simulink model "ProcNavNode"  (R2020a)
settings: Solver=FixedStepAuto  StartTime=0.0  StopTime=inf  FixedStep=.05  RelTol=1e-3
model workspace (MAT data in the model file):
  SL_ROS_VariableLengthArrays_MaxSizes.CommonInfo.ArrayTruncateAction = 'EmitWarning'
  SL_ROS_VariableLengthArrays_MaxSizes.MsgTypeMap = containers.Map
  SL_ROS_VariableLengthArrays_MaxSizes.MsgTypeMap.serialization.keys = {}
  SL_ROS_VariableLengthArrays_MaxSizes.MsgTypeMap.serialization.values = {}
  SL_ROS_VariableLengthArrays_MaxSizes.MsgTypeMap.serialization.uniformity = 0
  SL_ROS_VariableLengthArrays_MaxSizes.MsgTypeMap.serialization.keyType = 'char'
  SL_ROS_VariableLengthArrays_MaxSizes.MsgTypeMap.serialization.valueType = 'any'
libraries: robotlib x4
settings Model: SimulationMode=external  PauseTimes=1000  Creator=Lamarre  LastModifiedBy=lamarre
settings OptimizationCC: EnhancedBackFolding=on  PassReuseOutputArgsAs=Individual arguments  ZeroExternalMemoryAtStartup=off  ZeroInternalMemoryAtStartup=off  MaxStackSize=64  OptimizeBlockOrder=speed  DifferentSizesBufferReuse=on  OptimizationCustomize=off  EfficientTunableParamExpr=on
settings DebuggingCC: ParameterTunabilityLossMsg=error  FcnCallInpInsideContextMsg=warning  UnderSpecifiedDimensionMsg=warning
settings HardwareCC: ProdBitPerPointer=32  ProdBitPerSizeT=32  ProdBitPerPtrDiffT=32  ProdLargestAtomicInteger=Long  ProdWordSize=32  ProdHWDeviceType=ARM Compatible->ARM 8
settings ModelReferenceCC: ModelReferenceNumInstancesAllowed=Single
settings SFSimCC: MATLABDynamicMemAlloc=off
settings RTWCC: SystemTargetFile=ert.tlc  HardwareBoard=Robot Operating System (ROS)  TemplateMakefile=ert_default_tmf  Toolchain=Catkin  BuildConfiguration=Faster Runs  TargetLang=C++
settings CodeAppCC: ForceParamTrailComments=on  IgnoreCustomStorageClasses=off  OperatorAnnotations=on  SimulinkDataObjDesc=on  SFDataObjDesc=on  InsertBlockDesc=on
settings ERTTargetCC: MultiInstanceERTCode=on  CodeInterfacePackaging=C++ class  RootIOFormat=Structure reference

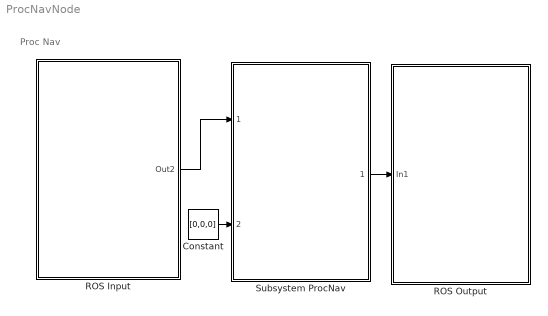
== system ProcNavNode ==
  note: Proc Nav
  Constant : Constant  Value=[0,0,0]
  ROS Input : Subsystem
  ROS Output : Subsystem
  Subsystem ProcNav : Subsystem  ReferencedSubsystem=ProcNav
  wires:
  ROS Input/1(Out2) -> Subsystem ProcNav/1
  Subsystem ProcNav/1 -> ROS Output/1(In1)
  Constant/1 -> Subsystem ProcNav/2

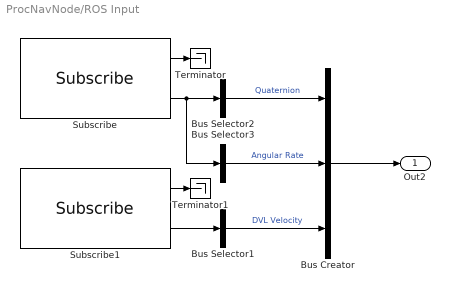
== system ProcNavNode/ROS Input ==
  Bus Creator : BusCreator  Inputs=3
  Bus Selector1 : BusSelector  OutputSignals=XVelBtm,YVelBtm,ZVelBtm  OutputAsBus=on
  Bus Selector2 : BusSelector  OutputSignals=Orientation.W,Orientation.X,Orientation.Y,Orientation.Z  OutputAsBus=on
  Bus Selector3 : BusSelector  OutputSignals=AngularVelocity.X,AngularVelocity.Y,AngularVelocity.Z  OutputAsBus=on
  Subscribe : robotlib/Subscribe  topicSource=Specify your own  topic=/provider_imu/imu_info  messageType=sensor_msgs/Imu  sampleTime=-1  messageQueueLength=1
  Subscribe1 : robotlib/Subscribe  topicSource=Specify your own  topic=/provider_dvl/dvl_velocity  messageType=sonia_common/BodyVelocityDVL  sampleTime=-1  messageQueueLength=1
  Terminator : Terminator
  Terminator1 : Terminator
  Out2 : Outport
  wires:
  Bus Selector3/1 -> Bus Creator/2  "Angular Rate"
  Bus Selector1/1 -> Bus Creator/3  "DVL Velocity"
  Bus Creator/1 -> Out2/1
  Subscribe1/1 -> Terminator1/1
  Subscribe/1 -> Terminator/1
  Bus Selector2/1 -> Bus Creator/1  "Quaternion"
  Subscribe/2 -> Bus Selector3/1, Bus Selector2/1
  Subscribe1/2 -> Bus Selector1/1

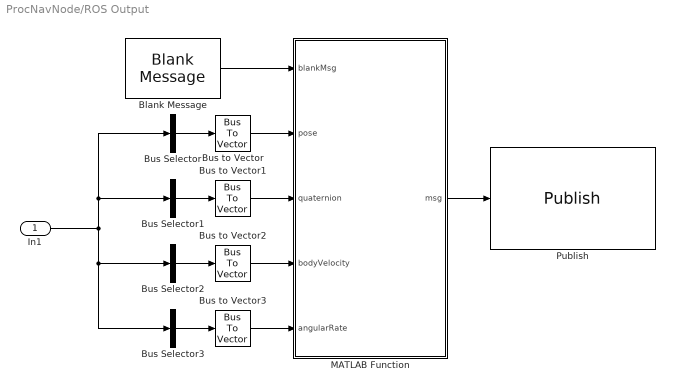
== system ProcNavNode/ROS Output ==
  In1 : Inport
  Blank Message : robotlib/Blank Message  messageClass=Message  entityType=sonia_common/ControllerStates  messageType=sonia_common/ControllerStates  SampleTime=inf
  Bus Selector : BusSelector  OutputSignals=World Position  OutputAsBus=on
  Bus Selector1 : BusSelector  OutputSignals=qS2W  OutputAsBus=on
  Bus Selector2 : BusSelector  OutputSignals=Body Velocity  OutputAsBus=on
  Bus Selector3 : BusSelector  OutputSignals=Angular Rate  OutputAsBus=on
  Bus to Vector{,1..3} (4 alike) : BusToVector
  MATLAB Function : MATLAB Function  TreatAsAtomicUnit=on
  Publish : robotlib/Publish  topicSource=Specify your own  topic=/proc_control/mesured_output  messageType=sonia_common/ControllerStates  messageQueueLength=1
  wires:
  Bus to Vector/1 -> MATLAB Function/2(pose)
  Bus to Vector2/1 -> MATLAB Function/4(bodyVelocity)
  Bus Selector2/1 -> Bus to Vector2/1
  Bus to Vector1/1 -> MATLAB Function/3(quaternion)
  In1/1 -> Bus Selector3/1, Bus Selector2/1, Bus Selector1/1, Bus Selector/1
  Blank Message/1 -> MATLAB Function/1(blankMsg)
  Bus Selector1/1 -> Bus to Vector1/1
  Bus to Vector3/1 -> MATLAB Function/5(angularRate)
  MATLAB Function/1(msg) -> Publish/1
  Bus Selector/1 -> Bus to Vector/1
  Bus Selector3/1 -> Bus to Vector3/1

== matlab function ProcNavNode/ROS Output/MATLAB Function ==
  data: blankMsg input; msg output SL_Bus_ProcNavNode_sonia_common_ControllerStates; pose input; quaternion input; bodyVelocity input; angularRate input
function msg = ControllerStateMsg(blankMsg,pose, quaternion, bodyVelocity, angularRate)
% assignStringInput - Assign a string in a ROS message to specified input string
%
% MSG = assignStringInput(blankMsg, STR) assigns the input string, STR, to
%  a string field in the ROS message, blankMsg, and outputs the updated
%  ROS message.
%
%  Inputs
%    blankMsg: A bus for a 'std_msgs/String' message. This is 
%        used to initialize the output.
%    str: An array of uint8 that will be assigned to the 'Data' field
%        in blankMsg. The entire array is assumed to be a valid sequence of
%        character ASCII values.
% 
%  Outputs:
%    msg: A bus for a 'std_msgs/String' message, with the 'Data'
%        field set to a string.

%   Copyright 2015 The MathWorks, Inc.
%#codegen

% Note: The datatype of 'msg' has been explicitly set to the appropriate 
% Simulink bus type ("Bus: SL_Bus_robotROSMessageUsageExample_std_msgs_String"). 
%
% If the model name is changed, the datatype needs to be changed as well:
%   1) Click "Edit Data" in the Editor toolstrip to open "Ports and Data Manager"
%   2) Select "msg". From the "Type" dropdown, select "--- Refresh data types ---"
%   3) Set datatype to "Bus: SL_Bus_<modelname>_std_msgs_String"
   
msg = blankMsg;


msg.Pose.Position.X = pose(1);
msg.Pose.Position.Y = pose(2);
msg.Pose.Position.Z = pose(3);

msg.Pose.Orientation.W = quaternion(1);
msg.Pose.Orientation.X = quaternion(2);
msg.Pose.Orientation.Y = quaternion(3);
msg.Pose.Orientation.Z = quaternion(4);

msg.Velocity.Linear.X = bodyVelocity(1);
msg.Velocity.Linear.Y = bodyVelocity(2);
msg.Velocity.Linear.Z = bodyVelocity(3);

msg.Velocity.Angular.X = angularRate(1);
msg.Velocity.Angular.Y =angularRate(2);
msg.Velocity.Angular.Z = angularRate(3);
